simulink model "s4"  (Simulink 2.00)
settings: Solver=ode15s  StartTime=0.0  StopTime=tstop  MaxStep=5e-3  RelTol=5e-6  AbsTol=1e-6
values from neighbouring files (symbols this model uses):
  delto = delt    [M1.M]    (also in M3.M; M4.M = 0; M5.M)
  Domega = 0    [M4.M]    (also in SET1.M; SET3A.M; SET3B.M; SET3C.M)
  H = 0.5*J_rotor*wbasem*wbasem/Sbase    [M1.M]    (also in M3.M; M4.M = 0.3; SET1.M = 3.77; SET3A.M = 3)
  Ipm = Emo/xmd    [M4.M]
  Psido = xls*(-Ido) + Psiado    [M1.M]    (also in M3.M; M4.M = Psiado; M5.M)
  Psikdo = Psiado    [M1.M]    (also in M3.M; M4.M)
  Psikqo = Psiaqo    [M1.M]    (also in M3.M; M4.M = 0)
  Psiqo = xls*(-Iqo) + Psiaqo    [M1.M]    (also in M3.M; M4.M = 0; M5.M)
  rpkd = rpkd/Zbase    [M1.M]    (also in M3.M; M4.M = 0.054)
  rpkq = rpkq/Zbase    [M1.M]    (also in M3.M; M4.M = 0.108)
  rs = rs/Zbase    [M1.M]    (also in M3.M; M4.M = 0.017; SET1.M = 0.0048; SET3A.M = 0.004)
  tmech_time = [0 tstop]    [M1.M]    (also in M4.M; M5.M)
  tmech_value = [1 1]*Tmech    [M1.M]    (also in M4.M = [-1 -1]*temo; M5.M)
  Vm = abs(Vt)    [M1.M]    (also in M3.M; M4.M; M5.M)
  wb = wbase    [M1.M]    (also in M3.M; M4.M = 376.991118431; M5.M)
  we = 2*pi*Frated    [M1.M]    (also in M3.M; M4.M = 376.991118431; M5.M)
  wrslipo = -1    [M4.M]
  xd = xd/Zbase    [M1.M]    (also in M3.M; M4.M = 0.543; SET1.M = 1.79; SET3A.M = 1.89)
  xls = xls/Zbase    [M1.M]    (also in M3.M; M4.M = 0.065; SET1.M = 0.215; SET3A.M = 0.19)
  xmd = xmd/Zbase    [M1.M]    (also in M3.M; M4.M = 0.478; SET3A.M = 1.7; SET3B.M = 1.7)
  xMD = (1/xls + 1/xmd + 1/xplf + 1/xplkd)^(-1)    [M1.M]    (also in M3.M; M4.M = 0.0399162984447; M5.M = (1/xls + 1/xmd + bsum)^(-1))
  xMQ = (1/xls + 1/xmq + 1/xplkq)^(-1)    [M1.M]    (also in M3.M; M4.M = 0.0417714348384; M5.M = (1/xls + 1/xmq + 1/xplkq3 + 1/xplkq2 + 1/xplkq1)^(-1))
  xplkd = xplkd/Zbase    [M1.M]    (also in M3.M; M4.M = 0.132)
  xplkq = xplkq/Zbase    [M1.M]    (also in M3.M; M4.M = 0.132)
  xq = xq/Zbase    [M1.M]    (also in M3.M; M4.M = 1.086; SET1.M = 1.66; SET3A.M = 1.8)
settings Model: SaveTime=off  SaveOutput=off  ConsistencyChecking=off

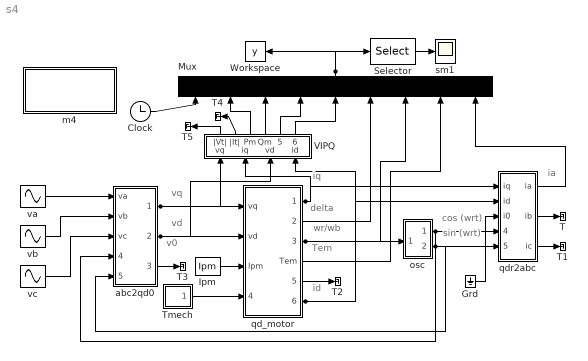
== system s4 ==
  note: vq
  note: v0
  note: wr/wb
  note: Tem
  note: cos (wrt)
  note: sin (wrt)
  note: vd
  note: id
  note: delta
  note: iq
  note: ia
  Clock : Clock
      settings: DeleteFcn=simclock BlockIsBeingDestroyed  PostSaveFcn=simclock Save
  Grd : Ground
  Ipm : Constant  Value=Ipm
  m4 : Subsystem
      settings: OpenFcn=m4
      mask Type: Masked block of m4.m
      mask Help: Uses m4.m to initialize and plot
      mask Display: disp('Initialize\nand plot')
  Mux : Mux  Orientation=up  Inputs=9
  Selector : Selector  Elements=[3 4 5 6 7 8]  InputPortWidth=9
  T{,1..5} (6 alike) : Terminator
  Tmech : Subsystem  mask(Repeating table){rep_seq_t=tmech_time, rep_seq_y=tmech_value}
      mask prompts: rep_seq_t "Time values:"; rep_seq_y "Output values:"
      mask help: Repeating table.
      mask init:
      | period = max(rep_seq_t);
      mask Help: Repeats cycle given in table. Time values should be monotonically increasing.
      mask Display: plot([rep_seq_t,rep_seq_t+period,rep_seq_t+2*period,rep_seq_t(1)+3*period],[rep_seq_y,rep_seq_y,rep_seq_y,rep_seq_y(1)])
  VIPQ : Subsystem  Orientation=up
  Workspace : ToWorkspace  VariableName=y  SampleTime=0
      settings: Buffer=100000
  abc2qd0 : Subsystem
  osc : Subsystem
  qd_motor : Subsystem
  qdr2abc : Subsystem
  sm1 : Scope
      settings: TickLabels=on  TimeRange=auto  YMin=-3  YMax=3  SaveToWorkspace=off  SaveName=ScopeData  LimitMaxRows=off
  va : Sin  Amplitude=Vm  Frequency=we  Phase=pi/2  SampleTime=-1
  vb : Sin  Amplitude=Vm  Frequency=we  Phase=-pi/6  SampleTime=-1
  vc : Sin  Amplitude=Vm  Frequency=we  Phase=7*pi/6  SampleTime=-1
  wires:
  vc/1 -> abc2qd0/3(vc)
  vb/1 -> abc2qd0/2(vb)
  va/1 -> abc2qd0/1(va)
  osc/1(cos_thetar) -> qdr2abc/4(cos_thetar), abc2qd0/4(cos_thetar)
  osc/2(sin_thetar) -> qdr2abc/5(sin_thetar), abc2qd0/5(sin_thetar)
  abc2qd0/1(vqr) -> qd_motor/1(vq), VIPQ/1(vq)
  qd_motor/1(iq_motor) -> qdr2abc/1(iq), VIPQ/2(iq)
  qd_motor/6(id_motor) -> qdr2abc/2(id), VIPQ/4(id)
  Tmech/1(out_1) -> qd_motor/4(Tmech)
  abc2qd0/2(vdr) -> qd_motor/2(vd), VIPQ/3(vd)
  VIPQ/3(Pm) -> Mux/2
  VIPQ/4(Qm) -> Mux/3
  Clock/1 -> Mux/1
  qdr2abc/1(ia) -> Mux/9
  qd_motor/4(Tem) -> Mux/8
  qd_motor/3(wr/wb) -> osc/1(wr/wb), Mux/7
  qd_motor/2(delta) -> Mux/6
  VIPQ/6(Texc) -> Mux/5
  VIPQ/5(Trel) -> Mux/4
  Ipm/1 -> qd_motor/3(Ipm)
  qdr2abc/2(ib) -> T/1
  qdr2abc/3(ic) -> T1/1
  qd_motor/5((wr-we)/wb) -> T2/1
  abc2qd0/3(vd0) -> T3/1
  Selector/1 -> sm1/1
  Mux/1 -> Workspace/1, Selector/1
  VIPQ/2(|It|) -> T4/1
  VIPQ/1(|Vt|) -> T5/1
  Grd/1 -> qdr2abc/3(i0)

== system s4/m4 ==
  note: Masked block of m4.m to
      | initialize s4.m and plot results

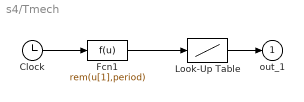
== system s4/Tmech ==
  Clock : Clock
      settings: DeleteFcn=simclock BlockIsBeingDestroyed  PostSaveFcn=simclock Save
  Fcn1 : Fcn  Expr=rem(u[1],period)
  Look-Up Table : Lookup  InputValues=rep_seq_t  OutputValues=rep_seq_y
  out_1 : Outport  Port=1  InitialOutput=0
  wires:
  Look-Up Table/1 -> out_1/1
  Clock/1 -> Fcn1/1
  Fcn1/1 -> Look-Up Table/1

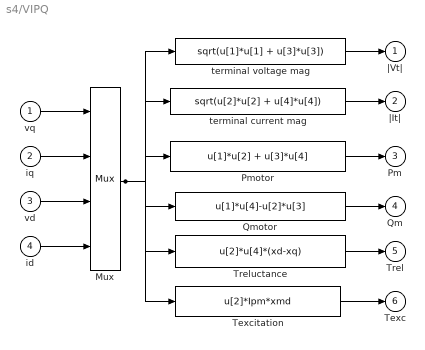
== system s4/VIPQ ==
  vq : Inport  Port=1  PortWidth=-1  SampleTime=-1
  iq : Inport  Port=2  PortWidth=-1  SampleTime=-1
  vd : Inport  Port=3  PortWidth=-1  SampleTime=-1
  id : Inport  Port=4  PortWidth=-1  SampleTime=-1
  Mux : Mux  Inputs=4
  Pmotor : Fcn  Expr=u[1]*u[2] + u[3]*u[4]
  Qmotor : Fcn  Expr=u[1]*u[4]-u[2]*u[3]
  Texcitation : Fcn  Expr=u[2]*Ipm*xmd
  "Treluctance " : Fcn  Expr=u[2]*u[4]*(xd-xq)
  terminal current mag : Fcn  Expr=sqrt(u[2]*u[2] + u[4]*u[4])
  terminal voltage mag : Fcn  Expr=sqrt(u[1]*u[1] + u[3]*u[3])
  |Vt| : Outport  Port=1  InitialOutput=0
  |It| : Outport  Port=2  InitialOutput=0
  Pm : Outport  Port=3  InitialOutput=0
  Qm : Outport  Port=4  InitialOutput=0
  Trel : Outport  Port=5  InitialOutput=0
  Texc : Outport  Port=6  InitialOutput=0
  wires:
  vq/1 -> Mux/1
  iq/1 -> Mux/2
  vd/1 -> Mux/3
  id/1 -> Mux/4
  Pmotor/1 -> Pm/1
  Qmotor/1 -> Qm/1
  Mux/1 -> Pmotor/1, Qmotor/1, terminal voltage mag/1, terminal current mag/1, "Treluctance "/1, Texcitation/1
  terminal voltage mag/1 -> |Vt|/1
  terminal current mag/1 -> |It|/1
  "Treluctance "/1 -> Trel/1
  Texcitation/1 -> Texc/1

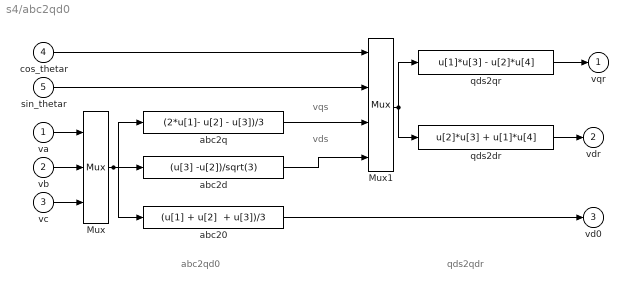
== system s4/abc2qd0 ==
  note: vds
  note: abc2qd0
  note: qds2qdr
  note: vqs
  va : Inport  Port=1  PortWidth=-1  SampleTime=-1
  vb : Inport  Port=2  PortWidth=-1  SampleTime=-1
  vc : Inport  Port=3  PortWidth=-1  SampleTime=-1
  cos_thetar : Inport  Port=4  PortWidth=-1  SampleTime=-1
  sin_thetar : Inport  Port=5  PortWidth=-1  SampleTime=-1
  Mux : Mux  Inputs=3
  Mux1 : Mux  Inputs=4
  abc20 : Fcn  Expr="(u[1] + u[2]  + u[3])/3"
  abc2d : Fcn  Expr=(u[3] -u[2])/sqrt(3)
  abc2q : Fcn  Expr=(2*u[1]- u[2] - u[3])/3
  qds2dr : Fcn  Expr=u[2]*u[3] + u[1]*u[4]
  qds2qr : Fcn  Expr=u[1]*u[3] - u[2]*u[4]
  vqr : Outport  Port=1  InitialOutput=0
  vdr : Outport  Port=2  InitialOutput=0
  vd0 : Outport  Port=3  InitialOutput=0
  wires:
  Mux/1 -> abc2q/1, abc2d/1, abc20/1
  Mux1/1 -> qds2qr/1, qds2dr/1
  va/1 -> Mux/1
  vb/1 -> Mux/2
  vc/1 -> Mux/3
  qds2qr/1 -> vqr/1
  qds2dr/1 -> vdr/1
  cos_thetar/1 -> Mux1/1
  sin_thetar/1 -> Mux1/2
  abc2q/1 -> Mux1/3
  abc2d/1 -> Mux1/4
  abc20/1 -> vd0/1

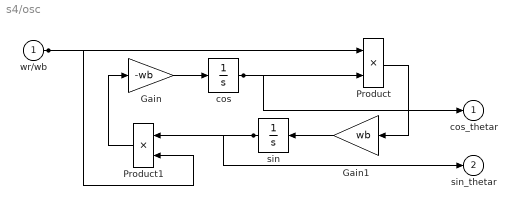
== system s4/osc ==
  wr/wb : Inport  Port=1  PortWidth=-1  SampleTime=-1
  Gain : Gain  Gain=-wb
  Gain1 : Gain  Orientation=left  Gain=wb
  Product : Product  Inputs=2
  Product1 : Product  Orientation=left  Inputs=2
  cos : Integrator  ExternalReset=none  InitialConditionSource=internal  InitialCondition=cos(delto)  LimitOutput=off  UpperSaturationLimit=inf  LowerSaturationLimit=-inf  ShowSaturationPort=off  ShowStatePort=off  AbsoluteTolerance=auto
  sin : Integrator  Orientation=left  ExternalReset=none  InitialConditionSource=internal  InitialCondition=sin(delto)  LimitOutput=off  UpperSaturationLimit=inf  LowerSaturationLimit=-inf  ShowSaturationPort=off  ShowStatePort=off  AbsoluteTolerance=auto
  cos_thetar : Outport  Port=1  InitialOutput=0
  sin_thetar : Outport  Port=2  InitialOutput=0
  wires:
  Product/1 -> Gain1/1
  cos/1 -> cos_thetar/1, Product/2
  Gain/1 -> cos/1
  Product1/1 -> Gain/1
  Gain1/1 -> sin/1
  wr/wb/1 -> Product/1, Product1/2
  sin/1 -> Product1/1, sin_thetar/1

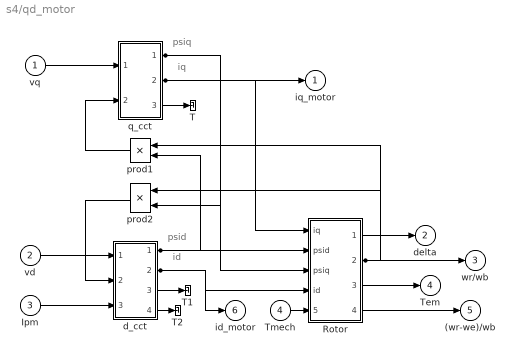
== system s4/qd_motor ==
  note: iq
  note: id
  note: psid
  note: psiq
  vq : Inport  Port=1  PortWidth=-1  SampleTime=-1
  vd : Inport  Port=2  PortWidth=-1  SampleTime=-1
  Ipm : Inport  Port=3  PortWidth=-1  SampleTime=-1
  Tmech : Inport  Port=4  PortWidth=-1  SampleTime=-1
  Rotor : Subsystem
  T : Terminator
  T1 : Terminator
  T2 : Terminator
  d_cct : Subsystem
  prod1 : Product  Orientation=left  Inputs=2
  prod2 : Product  Orientation=left  Inputs=2
  q_cct : Subsystem
  iq_motor : Outport  Port=1  InitialOutput=0
  delta : Outport  Port=2  InitialOutput=0
  wr/wb : Outport  Port=3  InitialOutput=0
  Tem : Outport  Port=4  InitialOutput=0
  (wr-we)/wb : Outport  Port=5  InitialOutput=0
  id_motor : Outport  Port=6  InitialOutput=0
  wires:
  Tmech/1 -> Rotor/5(Tmech)
  q_cct/2(Out_iq) -> Rotor/1(iq), iq_motor/1
  Rotor/1(delta) -> delta/1
  Rotor/4((wr-we)/wb) -> (wr-we)/wb/1
  Rotor/3(Tem) -> Tem/1
  d_cct/2(Out_id) -> Rotor/4(id), id_motor/1
  prod1/1 -> q_cct/2(In_wrpsid)
  vq/1 -> q_cct/1(In_vq)
  d_cct/1(Out_psid) -> Rotor/2("psid "), prod1/2
  Rotor/2("wr/wb ") -> wr/wb/1, prod1/1, prod2/1
  q_cct/1(Out_psiq) -> Rotor/3(psiq), prod2/2
  Ipm/1 -> d_cct/3(In_Ipm)
  vd/1 -> d_cct/1(In_vd)
  prod2/1 -> d_cct/2(In_wrpsiq)
  q_cct/3(Out_psimq) -> T/1
  d_cct/3(Out_psimd) -> T1/1
  d_cct/4(Out_iplkd) -> T2/1

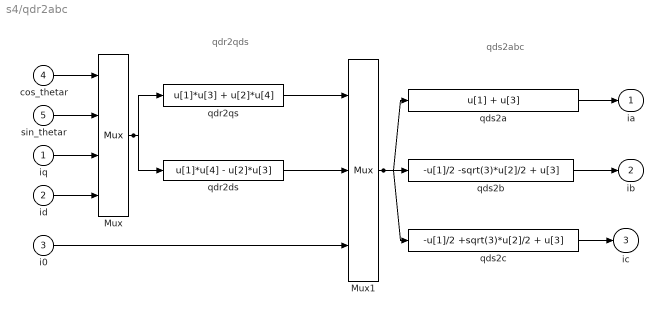
== system s4/qdr2abc ==
  note: qdr2qds
  note: qds2abc
  iq : Inport  Port=1  PortWidth=-1  SampleTime=-1
  id : Inport  Port=2  PortWidth=-1  SampleTime=-1
  i0 : Inport  Port=3  PortWidth=-1  SampleTime=-1
  cos_thetar : Inport  Port=4  PortWidth=-1  SampleTime=-1
  sin_thetar : Inport  Port=5  PortWidth=-1  SampleTime=-1
  Mux : Mux  Inputs=4
  Mux1 : Mux  Inputs=3
  qdr2ds : Fcn  Expr=u[1]*u[4] - u[2]*u[3]
  qdr2qs : Fcn  Expr=u[1]*u[3] + u[2]*u[4]
  qds2a : Fcn  Expr=u[1] + u[3]
  qds2b : Fcn  Expr=-u[1]/2 -sqrt(3)*u[2]/2 + u[3]
  qds2c : Fcn  Expr=-u[1]/2 +sqrt(3)*u[2]/2 + u[3]
  ia : Outport  Port=1  InitialOutput=0
  ib : Outport  Port=2  InitialOutput=0
  ic : Outport  Port=3  InitialOutput=0
  wires:
  cos_thetar/1 -> Mux/1
  sin_thetar/1 -> Mux/2
  iq/1 -> Mux/3
  id/1 -> Mux/4
  Mux/1 -> qdr2qs/1, qdr2ds/1
  qdr2qs/1 -> Mux1/1
  qdr2ds/1 -> Mux1/2
  i0/1 -> Mux1/3
  Mux1/1 -> qds2b/1, qds2a/1, qds2c/1
  qds2a/1 -> ia/1
  qds2b/1 -> ib/1
  qds2c/1 -> ic/1

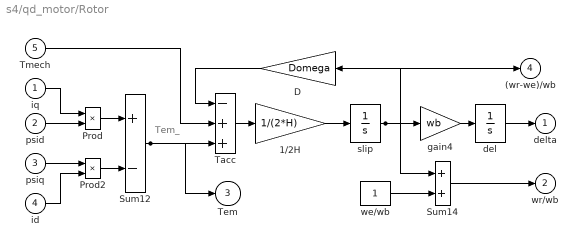
== system s4/qd_motor/Rotor ==
  note: Tem_
  iq : Inport  Port=1  PortWidth=-1  SampleTime=-1
  "psid " : Inport  Port=2  PortWidth=-1  SampleTime=-1
  psiq : Inport  Port=3  PortWidth=-1  SampleTime=-1
  id : Inport  Port=4  PortWidth=-1  SampleTime=-1
  Tmech : Inport  Port=5  PortWidth=-1  SampleTime=-1
  1/2H : Gain  Gain=1/(2*H)
  D : Gain  Orientation=left  Gain=Domega
  Prod : Product  Inputs=2
  Prod2 : Product  Inputs=2
  Sum12 : Sum  Inputs=+-
  Sum14 : Sum  Inputs=++
  Tacc : Sum  Inputs=-++
  del : Integrator  ExternalReset=none  InitialConditionSource=internal  InitialCondition=delto  LimitOutput=off  UpperSaturationLimit=inf  LowerSaturationLimit=-inf  ShowSaturationPort=off  ShowStatePort=off  AbsoluteTolerance=auto
  gain4 : Gain  Gain=wb
  slip : Integrator  ExternalReset=none  InitialConditionSource=internal  InitialCondition=wrslipo  LimitOutput=off  UpperSaturationLimit=inf  LowerSaturationLimit=-inf  ShowSaturationPort=off  ShowStatePort=off  AbsoluteTolerance=auto
  we/wb : Constant  Value=1
  delta : Outport  Port=1  InitialOutput=0
  "wr/wb " : Outport  Port=2  InitialOutput=0
  Tem : Outport  Port=3  InitialOutput=0
  (wr-we)/wb : Outport  Port=4  InitialOutput=0
  wires:
  D/1 -> Tacc/1
  gain4/1 -> del/1
  Prod2/1 -> Sum12/2
  1/2H/1 -> slip/1
  we/wb/1 -> Sum14/2
  Tacc/1 -> 1/2H/1
  Prod/1 -> Sum12/1
  iq/1 -> Prod/1
  "psid "/1 -> Prod/2
  psiq/1 -> Prod2/1
  id/1 -> Prod2/2
  Sum14/1 -> "wr/wb "/1
  Sum12/1 -> Tacc/3, Tem/1
  slip/1 -> gain4/1, Sum14/1, (wr-we)/wb/1, D/1
  Tmech/1 -> Tacc/2
  del/1 -> delta/1

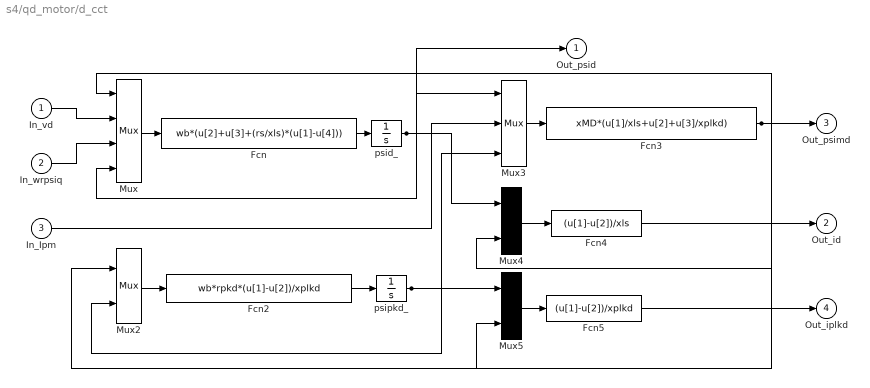
== system s4/qd_motor/d_cct ==
  In_vd : Inport  Port=1  PortWidth=-1  SampleTime=-1
  In_wrpsiq : Inport  Port=2  PortWidth=-1  SampleTime=-1
  In_Ipm : Inport  Port=3  PortWidth=-1  SampleTime=-1
  Fcn : Fcn  Expr=wb*(u[2]+u[3]+(rs/xls)*(u[1]-u[4]))
  Fcn2 : Fcn  Expr=wb*rpkd*(u[1]-u[2])/xplkd
  Fcn3 : Fcn  Expr=xMD*(u[1]/xls+u[2]+u[3]/xplkd)
  Fcn4 : Fcn  Expr=(u[1]-u[2])/xls
  Fcn5 : Fcn  Expr=(u[1]-u[2])/xplkd
  Mux : Mux  Inputs=4
  Mux2 : Mux  Inputs=2
  Mux3 : Mux  Inputs=3
  Mux4 : Mux  Inputs=2
  Mux5 : Mux  Inputs=2
  psid_ : Integrator  ExternalReset=none  InitialConditionSource=internal  InitialCondition=Psido  LimitOutput=off  UpperSaturationLimit=inf  LowerSaturationLimit=-inf  ShowSaturationPort=off  ShowStatePort=off  AbsoluteTolerance=auto
  psipkd_ : Integrator  ExternalReset=none  InitialConditionSource=internal  InitialCondition=Psikdo  LimitOutput=off  UpperSaturationLimit=inf  LowerSaturationLimit=-inf  ShowSaturationPort=off  ShowStatePort=off  AbsoluteTolerance=auto
  Out_psid : Outport  Port=1  InitialOutput=0
  Out_id : Outport  Port=2  InitialOutput=0
  Out_psimd : Outport  Port=3  InitialOutput=0
  Out_iplkd : Outport  Port=4  InitialOutput=0
  wires:
  In_wrpsiq/1 -> Mux/3
  In_vd/1 -> Mux/2
  Mux/1 -> Fcn/1
  Fcn/1 -> psid_/1
  Mux2/1 -> Fcn2/1
  Fcn2/1 -> psipkd_/1
  psid_/1 -> Mux/4, Mux3/1, Mux4/1, Out_psid/1
  psipkd_/1 -> Mux2/2, Mux3/3, Mux5/1
  Mux3/1 -> Fcn3/1
  Mux4/1 -> Fcn4/1
  Mux5/1 -> Fcn5/1
  Fcn3/1 -> Mux5/2, Mux4/2, Mux2/1, Mux/1, Out_psimd/1
  Fcn4/1 -> Out_id/1
  Fcn5/1 -> Out_iplkd/1
  In_Ipm/1 -> Mux3/2

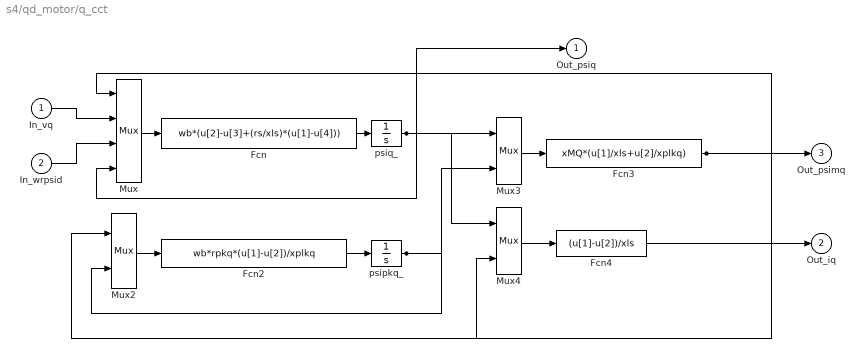
== system s4/qd_motor/q_cct ==
  In_vq : Inport  Port=1  PortWidth=-1  SampleTime=-1
  In_wrpsid : Inport  Port=2  PortWidth=-1  SampleTime=-1
  Fcn : Fcn  Expr=wb*(u[2]-u[3]+(rs/xls)*(u[1]-u[4]))
  Fcn2 : Fcn  Expr=wb*rpkq*(u[1]-u[2])/xplkq
  Fcn3 : Fcn  Expr=xMQ*(u[1]/xls+u[2]/xplkq)
  Fcn4 : Fcn  Expr=(u[1]-u[2])/xls
  Mux : Mux  Inputs=4
  Mux2 : Mux  Inputs=2
  Mux3 : Mux  Inputs=2
  Mux4 : Mux  Inputs=2
  psipkq_ : Integrator  ExternalReset=none  InitialConditionSource=internal  InitialCondition=Psikqo  LimitOutput=off  UpperSaturationLimit=inf  LowerSaturationLimit=-inf  ShowSaturationPort=off  ShowStatePort=off  AbsoluteTolerance=auto
  psiq_ : Integrator  ExternalReset=none  InitialConditionSource=internal  InitialCondition=Psiqo  LimitOutput=off  UpperSaturationLimit=inf  LowerSaturationLimit=-inf  ShowSaturationPort=off  ShowStatePort=off  AbsoluteTolerance=auto
  Out_psiq : Outport  Port=1  InitialOutput=0
  Out_iq : Outport  Port=2  InitialOutput=0
  Out_psimq : Outport  Port=3  InitialOutput=0
  wires:
  In_wrpsid/1 -> Mux/3
  In_vq/1 -> Mux/2
  Mux/1 -> Fcn/1
  Fcn/1 -> psiq_/1
  Mux2/1 -> Fcn2/1
  Fcn2/1 -> psipkq_/1
  psiq_/1 -> Mux/4, Mux3/1, Mux4/1, Out_psiq/1
  Mux3/1 -> Fcn3/1
  Mux4/1 -> Fcn4/1
  Fcn3/1 -> Mux4/2, Mux2/1, Mux/1, Out_psimq/1
  Fcn4/1 -> Out_iq/1
  psipkq_/1 -> Mux2/2, Mux3/2
